simulink model "hw2_p7"  (R2020a)
settings: Solver=VariableStepAuto  StartTime=0.0  StopTime=60  RelTol=1e-7
settings Model: Creator=Tomo  LastModifiedBy=Tomo

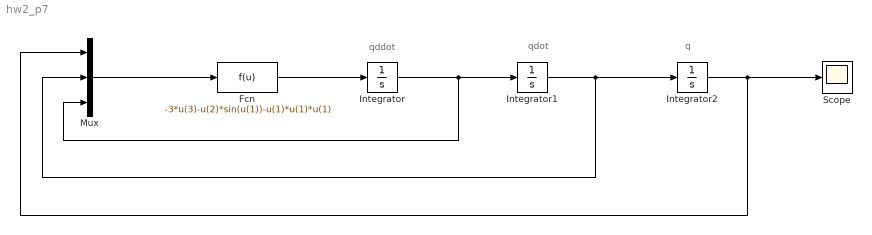
== system hw2_p7 ==
  note: q
  note: qdot
  note: qddot
  Fcn : Fcn  Expr=-3*u(3)-u(2)*sin(u(1))-u(1)*u(1)*u(1)
  Integrator : Integrator
  Integrator1 : Integrator
  Integrator2 : Integrator  InitialCondition=0.5
  Mux : Mux  Inputs=3
  Scope : Scope
  wires:
  Integrator2/1 -> Scope/1, Mux/1
  Integrator/1 -> Mux/3, Integrator1/1
  Integrator1/1 -> Integrator2/1, Mux/2
  Mux/1 -> Fcn/1
  Fcn/1 -> Integrator/1
